simulink library "INT_DrvDem_SelectParameter"  (R2016b)
settings: Solver=VariableStepAuto  StartTime=0.0  StopTime=10.0  RelTol=1e-3
settings Model: Creator=xuxingpei  LastModifiedBy=xuxingpei

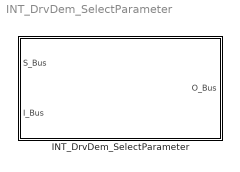
== system INT_DrvDem_SelectParameter ==
  INT_DrvDem_SelectParameter : Subsystem

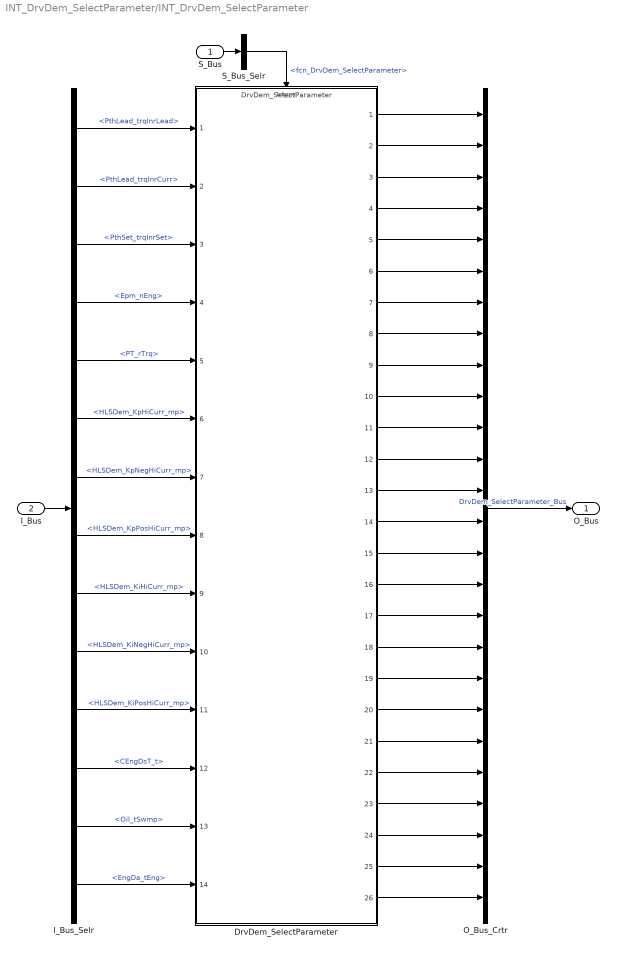
== system INT_DrvDem_SelectParameter/INT_DrvDem_SelectParameter ==
  S_Bus : Inport
  I_Bus : Inport  Port=2
  DrvDem_SelectParameter : ModelReference  ModelNameDialog=DrvDem_SelectParameter  SimulationMode=Normal  ModelReferenceVersion=1.41  TriggerPortName=function  TriggerPortTriggerType=function-call  TriggerPortStatesWhenEnabling=held
  I_Bus_Selr : BusSelector  OutputSignals=PthLead_trqInrLead,PthLead_trqInrCurr,PthSet_trqInrSet,Epm_nEng,PT_rTrq,HLSDem_KpHiCurr_mp,HLSDem_KpNegHiCurr_mp,HLSDem_KpPosHiCurr_mp,HLSDem_KiHiCurr_mp,HLSDem_KiNegHiCurr_mp,HLSDem_KiPosHiCurr_mp,CEngDsT_t,Oil_tSwmp,EngDa_tEng
  O_Bus_Crtr : BusCreator  Inputs=26
  S_Bus_Selr : BusSelector  OutputSignals=fcn_DrvDem_SelectParameter
  O_Bus : Outport
  wires:
  S_Bus_Selr/1 -> DrvDem_SelectParameter/Trigger  "<fcn_DrvDem_SelectParameter>"
  S_Bus/1 -> S_Bus_Selr/1
  I_Bus/1 -> I_Bus_Selr/1
  I_Bus_Selr/1 -> DrvDem_SelectParameter/1  "<PthLead_trqInrLead>"
  I_Bus_Selr/2 -> DrvDem_SelectParameter/2  "<PthLead_trqInrCurr>"
  I_Bus_Selr/3 -> DrvDem_SelectParameter/3  "<PthSet_trqInrSet>"
  I_Bus_Selr/4 -> DrvDem_SelectParameter/4  "<Epm_nEng>"
  I_Bus_Selr/5 -> DrvDem_SelectParameter/5  "<PT_rTrq>"
  I_Bus_Selr/6 -> DrvDem_SelectParameter/6  "<HLSDem_KpHiCurr_mp>"
  I_Bus_Selr/7 -> DrvDem_SelectParameter/7  "<HLSDem_KpNegHiCurr_mp>"
  I_Bus_Selr/8 -> DrvDem_SelectParameter/8  "<HLSDem_KpPosHiCurr_mp>"
  I_Bus_Selr/9 -> DrvDem_SelectParameter/9  "<HLSDem_KiHiCurr_mp>"
  I_Bus_Selr/10 -> DrvDem_SelectParameter/10  "<HLSDem_KiNegHiCurr_mp>"
  I_Bus_Selr/11 -> DrvDem_SelectParameter/11  "<HLSDem_KiPosHiCurr_mp>"
  I_Bus_Selr/12 -> DrvDem_SelectParameter/12  "<CEngDsT_t>"
  I_Bus_Selr/13 -> DrvDem_SelectParameter/13  "<Oil_tSwmp>"
  I_Bus_Selr/14 -> DrvDem_SelectParameter/14  "<EngDa_tEng>"
  O_Bus_Crtr/1 -> O_Bus/1  "DrvDem_SelectParameter_Bus"
  DrvDem_SelectParameter/1 -> O_Bus_Crtr/1
  DrvDem_SelectParameter/2 -> O_Bus_Crtr/2
  DrvDem_SelectParameter/3 -> O_Bus_Crtr/3
  DrvDem_SelectParameter/4 -> O_Bus_Crtr/4
  DrvDem_SelectParameter/5 -> O_Bus_Crtr/5
  DrvDem_SelectParameter/6 -> O_Bus_Crtr/6
  DrvDem_SelectParameter/7 -> O_Bus_Crtr/7
  DrvDem_SelectParameter/8 -> O_Bus_Crtr/8
  DrvDem_SelectParameter/9 -> O_Bus_Crtr/9
  DrvDem_SelectParameter/10 -> O_Bus_Crtr/10
  DrvDem_SelectParameter/11 -> O_Bus_Crtr/11
  DrvDem_SelectParameter/12 -> O_Bus_Crtr/12
  DrvDem_SelectParameter/13 -> O_Bus_Crtr/13
  DrvDem_SelectParameter/14 -> O_Bus_Crtr/14
  DrvDem_SelectParameter/15 -> O_Bus_Crtr/15
  DrvDem_SelectParameter/16 -> O_Bus_Crtr/16
  DrvDem_SelectParameter/17 -> O_Bus_Crtr/17
  DrvDem_SelectParameter/18 -> O_Bus_Crtr/18
  DrvDem_SelectParameter/19 -> O_Bus_Crtr/19
  DrvDem_SelectParameter/20 -> O_Bus_Crtr/20
  DrvDem_SelectParameter/21 -> O_Bus_Crtr/21
  DrvDem_SelectParameter/22 -> O_Bus_Crtr/22
  DrvDem_SelectParameter/23 -> O_Bus_Crtr/23
  DrvDem_SelectParameter/24 -> O_Bus_Crtr/24
  DrvDem_SelectParameter/25 -> O_Bus_Crtr/25
  DrvDem_SelectParameter/26 -> O_Bus_Crtr/26
